simulink model "Plant_Dynamic"  (R2020b)
settings: Solver=ode23  StartTime=0.0  StopTime=4  RelTol=1e-3
undefined symbols (not defined in the file): g, I_total_origin, m_total, X_com
settings Model: Creator=justi  LastModifiedBy=justi

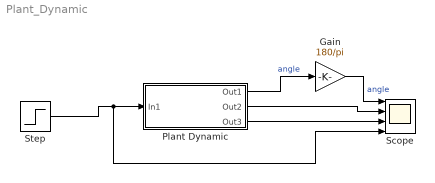
== system Plant_Dynamic ==
  Gain : Gain  Gain=180/pi
  Plant Dynamic : Subsystem
  Scope : Scope  NumInputPorts=4
  Step : Step  Time=5  After=0.04  SampleTime=0
  wires:
  Plant Dynamic/1(Out1) -> Gain/1  "angle"
  Step/1 -> Scope/4, Plant Dynamic/1(In1)
  Gain/1 -> Scope/1  "angle"
  Plant Dynamic/2(Out2) -> Scope/2
  Plant Dynamic/3(Out3) -> Scope/3

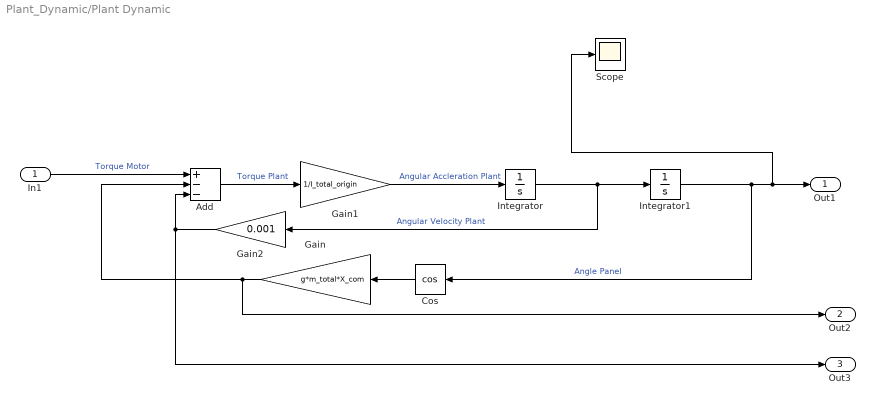
== system Plant_Dynamic/Plant Dynamic ==
  In1 : Inport
  Add : Sum  Inputs=+--
  Cos : Trigonometry  Operator=cos
  Gain : Gain  Gain=g*m_total*X_com
  Gain1 : Gain  Gain=1/I_total_origin
  Gain2 : Gain  Gain=0.001
  Integrator : Integrator
  Integrator1 : Integrator
  Scope : Scope
  Out1 : Outport
  Out2 : Outport  Port=2
  Out3 : Outport  Port=3
  wires:
  In1/1 -> Add/1  "Torque Motor"
  Cos/1 -> Gain/1
  Add/1 -> Gain1/1  "Torque Plant"
  Gain1/1 -> Integrator/1  "Angular Accleration Plant"
  Integrator/1 -> Gain2/1, Integrator1/1  "Angular Velocity Plant"
  Integrator1/1 -> Cos/1, Scope/1, Out1/1  "Angle Panel"
  Gain/1 -> Add/2, Out2/1
  Gain2/1 -> Add/3, Out3/1
